simulink model "SingleStreamSSR"  (R2020a)
settings: Solver=VariableStepAuto  StartTime=0.0  StopTime=4096  RelTol=1e-3
PreLoadFcn:
  | xmcCheckSlxPath(bdroot)
  | SSR4_init
undefined symbols (not defined in the file): FIR_MultiKernel_cin, FIR_MultiKernel_cincout, FIR_MultiKernel_cout, N, SHIFT_ACC, SingleStream, Taps, xc7vx485tffg1157
libraries: ModelComposer x37, dspsrcs4 x1, simulink x1
(part 1 of 3)
settings Model: Creator=oliviert  LastModifiedBy=abehbood

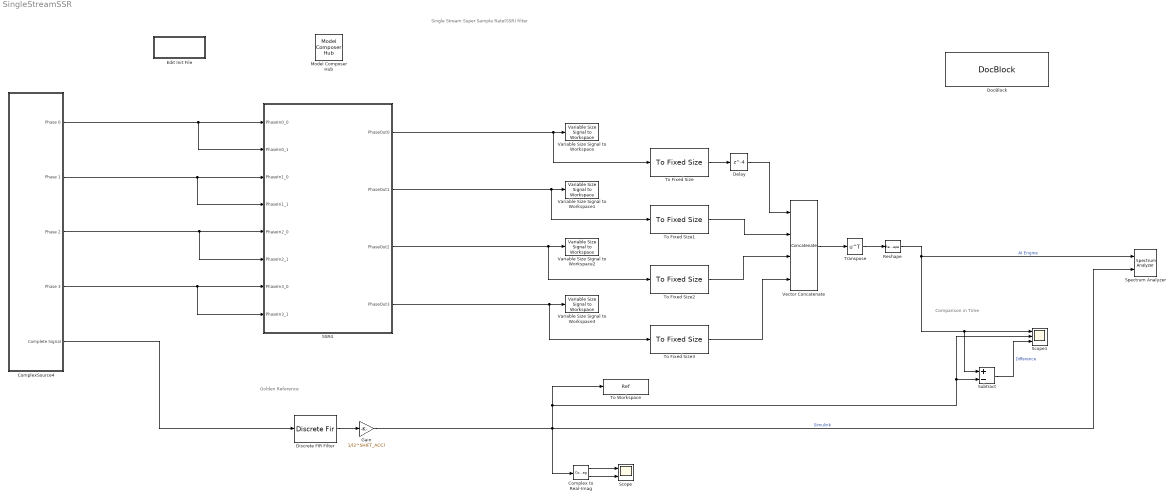
== system SingleStreamSSR ==
  note: Comparison in Time
  note: Golden Reference
  note: Single Stream Super Sample Rate(SSR) filter
  Complex to Real-Imag : ComplexToRealImag
  ComplexSource4 : Subsystem  mask{s=0}
      mask prompts: s "Seed"
  Delay : Delay  DelayLength=4  InputProcessing=Columns as channels (frame based)
  Discrete FIR Filter : DiscreteFir  Coefficients=Taps  InputProcessing=Columns as channels (frame based)
  DocBlock : simulink/Model-Wide Utilities/DocBlock  DocumentType=Text  mask(DocBlock){}
      content=|
      | ///////////////////////////////////////////////////////////////////////////
      | // Copyright 2021 Xilinx
      | //
      | // Licensed under the Apache License, Version 2.0 (the "License");
      | // you may not use this file except in compliance with the License.
      | // You may obtain a copy of the License at
      | //
      | // http://www.apache.org/licenses/LICENSE-2.0
      | //
      | // Unless required by applicable law or agreed to in writing, software
      | // distributed under the License is distributed on an "AS IS" BASIS,
      | // WITHOUT WARRANTIES OR CONDITIONS OF ANY KIND, either express or implied.
      | // See the License for the specific language governing permissions and
      | // limitations under the License.
      | ///////////////////////////////////////////////////////////////////////////
      mask Display:
      | xmcDrawBlockIcon();
      | disp(['{\fontsize{10pt}(c) Copyright 2021' ' Xilinx, Inc.}\newline \newline '],'texmode','on');
      | disp('{\fontsize{10pt}Licensed under the Apache License 2.0}','texmode','on');
      | disp('\newline \newline \newline{\fontsize{10pt}Double Click for Copyright Notice}','texmode','on');
  Edit Init File : Subsystem
      settings: OpenFcn=edit('SSR4_init.m');
  Gain : Gain  Gain=1/(2^SHIFT_ACC)
  Model Composer Hub : ModelComposer/Model Composer Hub  CodeGeneration=off  SubsystemName=SSR4  TargetDirectory=./code  ExportType=AI Engines  IpVendor=xilinx.com  IpLibrary=hls  IpVersion=1.0  IpHWLanguage=Verilog  AieCompilerOptions={}  CreateTestbench=on  TestbenchStackSize=10  RunAieSim=on  AieSimTimeout=5000  RunAieSimProfiling=off  LaunchVitisAnalyzer=on  PlotOutput=off  RunX86Sim=off  X86SimTimeout=10  GenHwImage=off  PlatformType=Not Specified  ProjDevice=xc7vx485tffg1157-1  ProjDevicePart=xc7vx485tffg1157-1  SamplePeriod=-1  ClockFrequency=200  DataPathParallelism=1
  Reshape : Reshape
  SSR4 : Subsystem
  Scope : Scope  NumInputPorts=2
  Scope1 : Scope  NumInputPorts=3
  Spectrum Analyzer : SpectrumAnalyzer  NumInputPorts=2
  Subtract : Sum  Inputs=+-
  To Fixed Size{,1..3} (4 alike) : ModelComposer/To Fixed Size  CopyMethod=Pad with zeros or discard excess samples  HasStatusOutput=off  OutputSizeCheck=on  OutputSize=N
  To Workspace : ToWorkspace  VariableName=Ref  SampleTime=-1
      settings: Save2DSignal=2-D array (concatenate along first dimension)
  Transpose : Math  Operator=transpose  SaturateOnIntegerOverflow=on
  Variable Size Signal to Workspace : ModelComposer/Variable Size Signal to Workspace  VariableNameMask=P0
  Variable Size Signal to Workspace1 : ModelComposer/Variable Size Signal to Workspace  VariableNameMask=P1
  Variable Size Signal to Workspace2 : ModelComposer/Variable Size Signal to Workspace  VariableNameMask=P2
  Variable Size Signal to Workspace3 : ModelComposer/Variable Size Signal to Workspace  VariableNameMask=P3
  Vector Concatenate : Concatenate  NumInputs=4  Mode=Multidimensional array  ConcatenateDimension=2
  wires:
  SSR4/2(PhaseOut1) -> To Fixed Size1/1, Variable Size Signal to Workspace1/1
  Complex to Real-Imag/2 -> Scope/2
  To Fixed Size1/1 -> Vector Concatenate/2
  Reshape/1 -> Subtract/1, Scope1/1, Spectrum Analyzer/1  "AI Engine"
  ComplexSource4/2(Phase 1) -> SSR4/4(PhaseIn1_1), SSR4/3(PhaseIn1_0)
  Complex to Real-Imag/1 -> Scope/1
  SSR4/1(PhaseOut0) -> To Fixed Size/1, Variable Size Signal to Workspace/1
  Subtract/1 -> Scope1/3  "Difference"
  ComplexSource4/1(Phase 0) -> SSR4/2(PhaseIn0_1), SSR4/1(PhaseIn0_0)
  Vector Concatenate/1 -> Transpose/1
  To Fixed Size3/1 -> Vector Concatenate/4
  ComplexSource4/3(Phase 2) -> SSR4/6(PhaseIn2_1), SSR4/5(PhaseIn2_0)
  To Fixed Size2/1 -> Vector Concatenate/3
  Transpose/1 -> Reshape/1
  Delay/1 -> Vector Concatenate/1
  ComplexSource4/4(Phase 3) -> SSR4/8(PhaseIn3_1), SSR4/7(PhaseIn3_0)
  ComplexSource4/5(Complete Signal) -> Discrete FIR Filter/1
  Discrete FIR Filter/1 -> Gain/1
  SSR4/3(PhaseOut2) -> To Fixed Size2/1, Variable Size Signal to Workspace2/1
  Gain/1 -> Spectrum Analyzer/2, Subtract/2, Scope1/2, To Workspace/1, Complex to Real-Imag/1  "Simulink"
  To Fixed Size/1 -> Delay/1
  SSR4/4(PhaseOut3) -> To Fixed Size3/1, Variable Size Signal to Workspace3/1

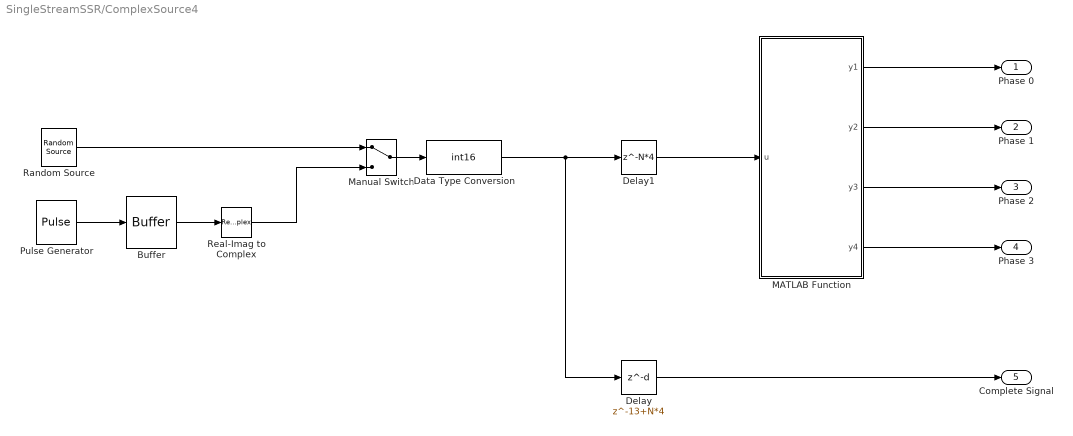
== system SingleStreamSSR/ComplexSource4 ==
  Buffer : Buffer  N=N*4  OutputFrames=off
  Data Type Conversion : DataTypeConversion  OutDataTypeStr=int16
  Delay : Delay  DelayLength=13+N*4  InputProcessing=Columns as channels (frame based)
  Delay1 : Delay  DelayLength=N*4  InputProcessing=Columns as channels (frame based)
  MATLAB Function : MATLAB Function  TreatAsAtomicUnit=on
  Manual Switch : ManualSwitch
  Pulse Generator : DiscretePulseGenerator  Amplitude=20000  Period=32 + 40*5  PhaseDelay=32  SampleTime=1/8
  Random Source : dspsrcs4/Random Source  SrcType=Uniform  NormMethod=Ziggurat  CltLength=12  MinVal=-20000  MaxVal=20000  MeanVal=0  VarVal=1  RepMode=Specify seed  rawSeed=s  IsInherit=off  SampMode=Discrete  SampTime=1/8  SampFrame=4*N  DataType=Double  OutComplex=Complex  OutputFrames=off
  Real-Imag to Complex : RealImagToComplex  Input=Real
  Phase 0 : Outport
  Phase 1 : Outport  Port=2
  Phase 2 : Outport  Port=3
  Phase 3 : Outport  Port=4
  Complete Signal : Outport  Port=5
  wires:
  MATLAB Function/1(y1) -> Phase 0/1
  MATLAB Function/2(y2) -> Phase 1/1
  MATLAB Function/3(y3) -> Phase 2/1
  MATLAB Function/4(y4) -> Phase 3/1
  Real-Imag to Complex/1 -> Manual Switch/2
  Pulse Generator/1 -> Buffer/1
  Delay/1 -> Complete Signal/1
  Buffer/1 -> Real-Imag to Complex/1
  Manual Switch/1 -> Data Type Conversion/1
  Random Source/1 -> Manual Switch/1
  Data Type Conversion/1 -> Delay1/1, Delay/1
  Delay1/1 -> MATLAB Function/1(u)

== system SingleStreamSSR/Edit Init File ==
